simulink model "POSTRG"  (R2022b)
settings: configuration reference "SharedConfig" (kept outside this file)
values from neighbouring files (symbols this model uses):
  MotPosnTrigDialEna_C = 0.0    [POSTRG.sldd]
  MotPosnTrigDialVal_CA : value not decoded    [POSTRG.sldd]
undefined symbols (not defined in the file or in its folder): slcm
Description:
  | Performs the trig calculations on the motor position that are used by the reference frame transforms.
settings Model: DataDictionary=POSTRG.sldd  Creator=Kevin  LastModifiedBy=Max Kolesnikov
settings ConfigSetRef: SourceName=SharedConfig

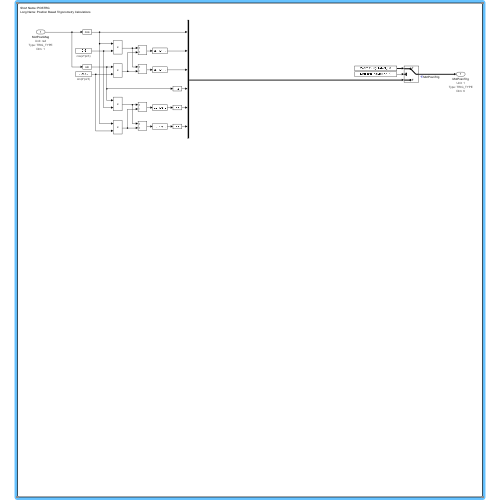
[thumbnail: Simulink's stored preview of the top-level diagram]
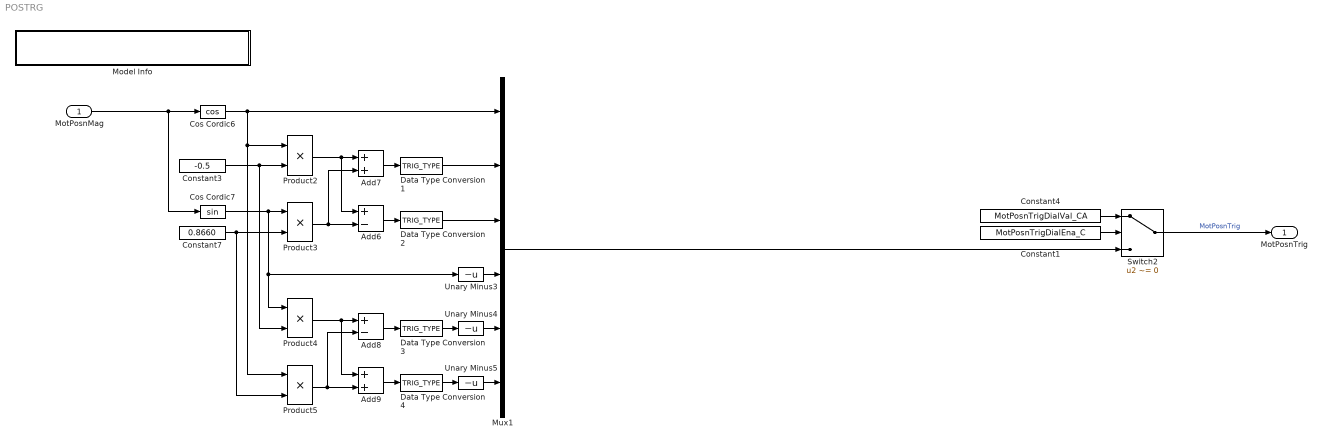
== system POSTRG ==
  MotPosnMag : Inport  OutDataTypeStr=TRIG_TYPE  Unit=rad  PortDimensions=1
      settings: AttributesFormatString=|
      | Unit: %<Unit>
      | Type: %<OutDataTypeStr>
      | Dim: %<PortDimensions>
  Add6 : Sum  Inputs=+-
  Add7 : Sum
  Add8 : Sum  Inputs=+-
  Add9 : Sum
  Constant1 : Constant  Value=MotPosnTrigDialEna_C
  Constant3 : Constant  Description=cos(2*pi/3)  Value=-0.5  OutDataTypeStr=TRIG_TYPE
      settings: AttributesFormatString=%<Description>
  Constant4 : Constant  Value=MotPosnTrigDialVal_CA
  Constant7 : Constant  Description=sin(2*pi/3)  Value=0.8660  OutDataTypeStr=TRIG_TYPE
      settings: AttributesFormatString=%<Description>
  Cos Cordic6 : Trigonometry  Operator=cos  NumberOfIterations=5
  Cos Cordic7 : Trigonometry  NumberOfIterations=5
  Data Type Conversion{1..4} (4 alike) : DataTypeConversion  OutDataTypeStr=TRIG_TYPE  SaturateOnIntegerOverflow=off  RndMeth=Floor
  Model Info : Subsystem  LoadFcn=slcm LoadBlock;  InitFcn=slcm('UpdateAllCMBlocksInThisModelInit')  mask(CMBlock){Frame=off, DisplayStringWithTags=|, MaskDisplayString=Short Name: POSTRG\nLong Name: Position Based Trigonometry Calculations, HorizontalTextAlignment=Left, LeftAlignmentValue=0.02}
      mask DisplayStringWithTags=|
      | Short Name: %<ModelName>
      | Long Name: Position Based Trigonometry Calculations
      mask prompts: Frame "Simulink:masks:Frame_MP"; DisplayStringWithTags "Simulink:masks:DisplayStringWithTags_MP"; MaskDisplayString "Simulink:masks:MaskDisplayString_MP"; HorizontalTextAlignment "Simulink:masks:HorizontalTextAlignment_MP"; LeftAlignmentValue "Simulink:masks:LeftAlignmentValue_MP"
      mask help: Simulink:masks:CMBlock_MD
      settings: CopyFcn=slcm CopyBlock;  DeleteFcn=slcm Cancel;  PostSaveFcn=slcm('UpdateAllCMBlocksInThisModel')  NameChangeFcn=slcm Rename;  OpenFcn=slcm
      mask Display: text(slResolve(LeftAlignmentValue, gcbh), 0.5, MaskDisplayString, 'HorizontalAlignment', HorizontalTextAlignment)
  Mux1 : Mux  Inputs=6
  Product{2..5} (4 alike) : Product
  Switch2 : Switch  Criteria=u2 ~= 0  SaturateOnIntegerOverflow=off  InputSameDT=off
  Unary Minus3 : UnaryMinus
  Unary Minus4 : UnaryMinus
  Unary Minus5 : UnaryMinus
  MotPosnTrig : Outport  OutDataTypeStr=TRIG_TYPE  Unit=1  PortDimensions=6
      settings: AttributesFormatString=|
      | Unit: %<Unit>
      | Type: %<OutDataTypeStr>
      | Dim: %<PortDimensions>
  wires:
  MotPosnMag/1 -> Cos Cordic7/1, Cos Cordic6/1
  Cos Cordic6/1 -> Mux1/1, Product5/1, Product2/1
  Cos Cordic7/1 -> Product4/1, Unary Minus3/1, Product3/1
  Constant3/1 -> Product4/2, Product2/2
  Product2/1 -> Add6/1, Add7/1
  Product3/1 -> Add7/2, Add6/2
  Constant7/1 -> Product5/2, Product3/2
  Add7/1 -> Data Type Conversion1/1
  Add6/1 -> Data Type Conversion2/1
  Unary Minus3/1 -> Mux1/4
  Unary Minus4/1 -> Mux1/5
  Unary Minus5/1 -> Mux1/6
  Add8/1 -> Data Type Conversion3/1
  Product4/1 -> Add9/1, Add8/1
  Product5/1 -> Add8/2, Add9/2
  Add9/1 -> Data Type Conversion4/1
  Switch2/1 -> MotPosnTrig/1  "MotPosnTrig"
  Data Type Conversion1/1 -> Mux1/2
  Data Type Conversion2/1 -> Mux1/3
  Data Type Conversion3/1 -> Unary Minus4/1
  Data Type Conversion4/1 -> Unary Minus5/1
  Constant1/1 -> Switch2/2
  Constant4/1 -> Switch2/1
  Mux1/1 -> Switch2/3

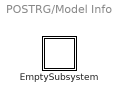
== system POSTRG/Model Info ==
  EmptySubsystem : Subsystem

== system POSTRG/Model Info/EmptySubsystem ==
